simulink model "softarm_tendon_force_demo"  (R2025a)
settings: Solver=ode15s  StartTime=0.0  StopTime=0.5  RelTol=1e-3
PreLoadFcn:
  | softarm_model_dir=fileparts(get_param(bdroot,'FileName'));softarm_root=fileparts(fileparts(softarm_model_dir));addpath(fullfile(softarm_root,'matlab'));addpath(fullfile(softarm_root,'matlab','simulink'));
InitFcn:
  | softarm_model_dir=fileparts(get_param(bdroot,'FileName'));softarm_root=fileparts(fileparts(softarm_model_dir));addpath(fullfile(softarm_root,'matlab'));addpath(fullfile(softarm_root,'matlab','simulink'));softarm_plant_block=string(bdroot)+"/Plant";softarm.applyPlantMask(softarm_plant_block,'force');
undefined symbols (not defined in the file): softarm_nq, softarm_u0, softarm_x0
settings Model: Creator=rlwan  LastModifiedBy=rlwan
settings DataIOCC: ReturnWorkspaceOutputs=off

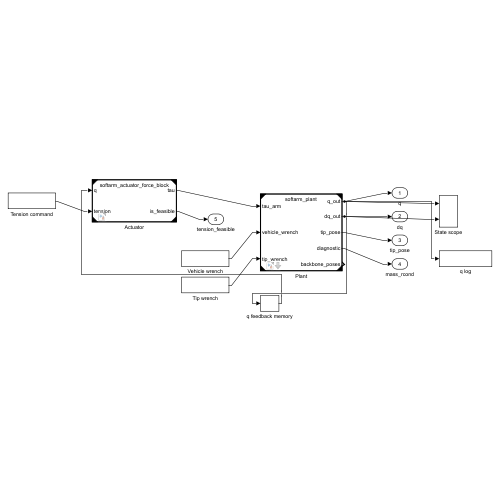
[thumbnail: Simulink's stored preview of the top-level diagram]
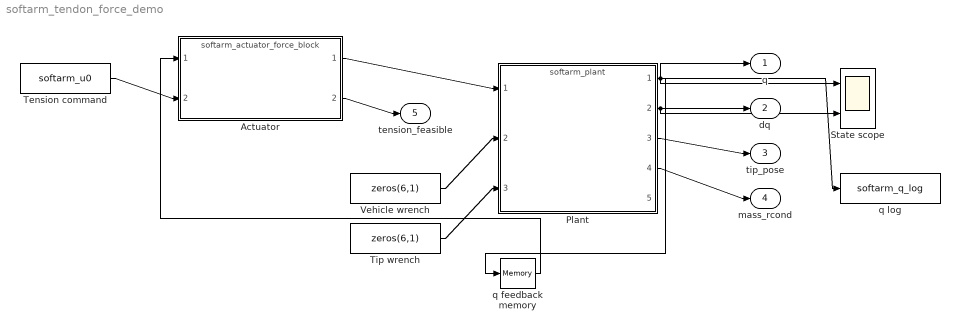
== system softarm_tendon_force_demo ==
  Actuator : ModelReference  ModelNameDialog=softarm_actuator_force_block  ModelReferenceVersion=1.1
  Plant : ModelReference  ModelNameDialog=softarm_plant  ParameterArgumentNames=Bundle  ParameterArgumentValues=Bundle  UsingDefaultArgumentValue=0  ModelReferenceVersion=1.1  Bundle='../generated/extensible_kirchhoff_pcs_three_tendon_n2'
  State scope : Scope  NumInputPorts=2
  Tension command : Constant  Value=softarm_u0
  Tip wrench : Constant  Value=zeros(6,1)
  Vehicle wrench : Constant  Value=zeros(6,1)
  q feedback memory : Memory  InitialCondition=softarm_x0(1:softarm_nq)
  q log : ToWorkspace  VariableName=softarm_q_log  SaveFormat=Timeseries  SampleTime=-1
  q : Outport
  dq : Outport  Port=2
  tip_pose : Outport  Port=3
  mass_rcond : Outport  Port=4
  tension_feasible : Outport  Port=5
  wires:
  Plant/1 -> q log/1, q feedback memory/1, q/1, State scope/1
  Tension command/1 -> Actuator/2
  Actuator/1 -> Plant/1
  Actuator/2 -> tension_feasible/1
  Vehicle wrench/1 -> Plant/2
  Tip wrench/1 -> Plant/3
  q feedback memory/1 -> Actuator/1
  Plant/2 -> dq/1, State scope/2
  Plant/3 -> tip_pose/1
  Plant/4 -> mass_rcond/1
